simulink model "MPC_of_Car"  (R2021b)
settings: Solver=VariableStepAuto  StartTime=0.0  StopTime=10.0  RelTol=1e-3
libraries: mpclib x1, cstblocks x1
settings Model: Creator=manavbathija  LastModifiedBy=manavbathija

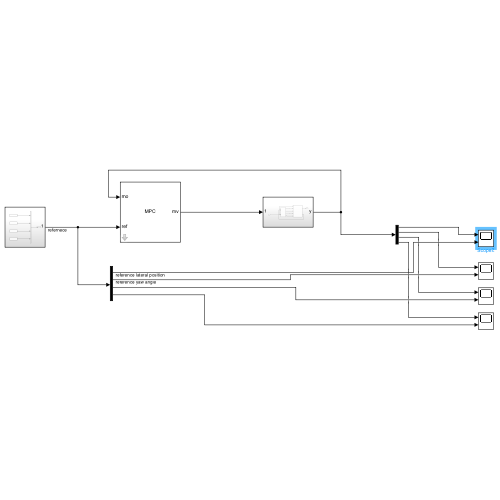
[thumbnail: Simulink's stored preview of the top-level diagram]
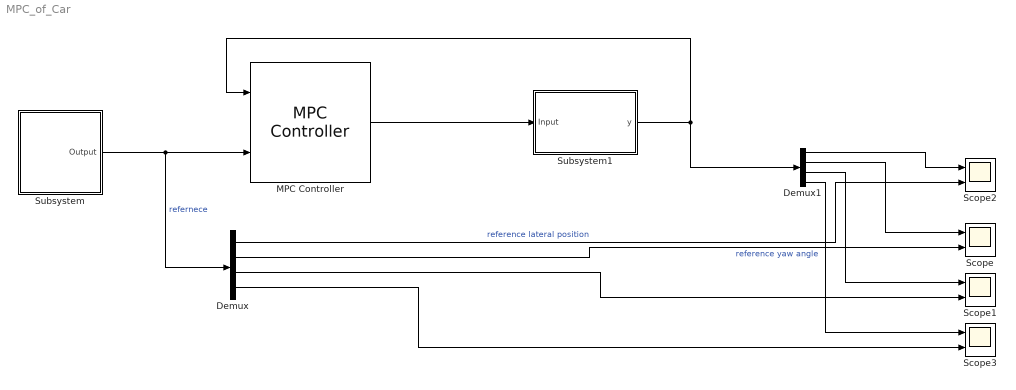
== system MPC_of_Car ==
  Demux : Demux
  Demux1 : Demux
  MPC Controller : mpclib/MPC Controller  SCDEnableBlockLinearizationSpecification=on  mpcobj=mpc1  is_multiple=0  enable_value=0  return_u0=off  updateMPCinCallerWorkspace=on  md_inport=off  mv_inport=off  uref_inport=off  return_cost=off  return_mvseq=off  return_qpstatus=off  return_xseq=off  return_state=off  return_ovseq=off  state_inport=off  umin_inport=off  umax_inport=off  ymin_inport=off  ymax_inport=off  cc_inport=off  ywt_inport=off  uwt_inport=off  duwt_inport=off  rhoeps_inport=off  pm_inport=off  MaximumP=10  HorizonChoice=FixedHorizon  n_ts=0.1  n_p=8  n_mv=2  n_md=0  n_ud=0  n_mo=4  n_uo=0  BlockDataType=double  SampleTimeInherited=off  switch_inport=off
  Scope{,1..3} (4 alike) : Scope  NumInputPorts=2
  Subsystem : Subsystem
  Subsystem1 : Subsystem
  wires:
  Subsystem/1(Output) -> MPC Controller/2, Demux/1  "refernece"
  MPC Controller/1 -> Subsystem1/1(Input)
  Subsystem1/1(y) -> MPC Controller/1, Demux1/1
  Demux/2 -> Scope/2  "reference yaw angle"
  Demux/3 -> Scope1/2
  Demux1/2 -> Scope/1
  Demux1/3 -> Scope1/1
  Demux1/1 -> Scope2/1
  Demux1/4 -> Scope3/1
  Demux/1 -> Scope2/2  "reference lateral position"
  Demux/4 -> Scope3/2

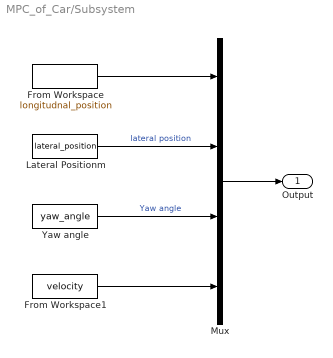
== system MPC_of_Car/Subsystem ==
  From Workspace : FromWorkspace  VariableName=longitudnal_position
  From Workspace1 : FromWorkspace  VariableName=velocity
  Lateral Positionm : FromWorkspace  VariableName=lateral_position
  Mux : Mux
  Yaw angle : FromWorkspace  VariableName=yaw_angle
  Output : Outport
  wires:
  Mux/1 -> Output/1
  Yaw angle/1 -> Mux/3  "Yaw angle"
  Lateral Positionm/1 -> Mux/2  "lateral position"
  From Workspace/1 -> Mux/1
  From Workspace1/1 -> Mux/4

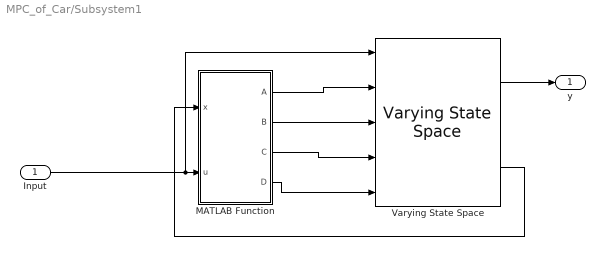
== system MPC_of_Car/Subsystem1 ==
  Input : Inport
  MATLAB Function : MATLAB Function  TreatAsAtomicUnit=on
  Varying State Space : cstblocks/Linear Parameter Varying/Varying State Space  x0=initial_state  xNames=''  OutputX=on  OutputDX=off
  y : Outport
  wires:
  Varying State Space/1 -> y/1
  MATLAB Function/3(C) -> Varying State Space/4
  MATLAB Function/4(D) -> Varying State Space/5
  Varying State Space/2 -> MATLAB Function/1(x)
  MATLAB Function/2(B) -> Varying State Space/3
  MATLAB Function/1(A) -> Varying State Space/2
  Input/1 -> Varying State Space/1, MATLAB Function/2(u)

== matlab function MPC_of_Car/Subsystem1/MATLAB Function ==
  data: x input; u input; A output; B output; C output; D output
function [A,B,C,D] = fcn(x,u)
    % The ego car has rectangular shaper with a length of 5 meters and width of
    % 2 meters. The model has four states:
    %
    % * |xPos| - Global horizontal position of the car center
    % * |yPos| - Global vertical position of the car center
    % * |theta| - Heading angle of the car (0 when facing east, counterclockwise positive)
    % * |V| - Speed of the car (positve)
    %
    % There are two manipulated variables:
    %
    % * |throttle| - Throttle (positive when accelerating, negative when braking)
    % * |delta| - Steering angle change (counterclockwise positive)
    
    %#codegen
    
    % Define continuous-time linear model from Jacobian of the nonlinear model.
    carLength = 5;
    theta = x(3);
    V = x(4);
    delta=u(2);
    A = [ 0, 0, -V*sin(theta), cos(theta);
           0, 0,  V*cos(theta), sin(theta);
           0, 0, 0,tan(delta)/carLength;
           0, 0, 0,0];
    B = [0  , 0;
          0  , 0;
          0  , (V*(tan(delta)^2 + 1))/carLength;
          0.5, 0];
    C= eye(4);
    D = zeros(4,2);
end
